simulink model "mdlref_paramargs"  (Simulink 6.0)
settings: Solver=FixedStepDiscrete  SolverMode=SingleTasking  StartTime=0.0  StopTime=10.0  FixedStep=0.1  RelTol=1e-3
undefined symbols (not defined in the file or in its folder): lower_saturation_limit, upper_saturation_limit
settings Model: Creator=The MathWorks Inc.  LastModifiedBy=batserve  ExtModeAutoUpdateStatusClock=off  ProdHWDeviceType=Specified
settings DataIOCC: SaveFormat=StructureWithTime  SignalLoggingName=logsOut
settings OptimizationCC: InlineParams=on
settings DebuggingCC: CheckExecutionContextPreStartOutputMsg=on  CheckExecutionContextRuntimeOutputMsg=on  SolverPrmCheckMsg=none
settings HardwareCC: ProdHWDeviceType=Specified  TargetHWDeviceType=32-bit Generic  ProdEqTarget=off
settings ModelReferenceCC: UpdateModelReferenceTargets=IfOutOfDate  CheckModelReferenceTargetMessage=none
settings RTWCC: GenerateReport=on  ProcessScript=grt_make_rtw_hook  LaunchReport=on

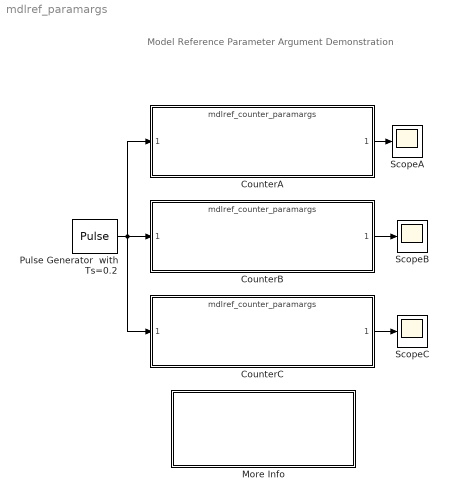
== system mdlref_paramargs ==
  note: Model Reference
      | Parameter Argument
      | Demonstration
  CounterA : ModelReference  ModelName=mdlref_counter_paramargs  ParameterArgumentNames=lower_saturation_limit,upper_saturation_limit  ParameterArgumentValues=0,20  ModelReferenceVersion=1.97  CopyOfModelName=mdlref_counter_paramargs
  CounterB : ModelReference  ModelName=mdlref_counter_paramargs  ParameterArgumentNames=lower_saturation_limit,upper_saturation_limit  ParameterArgumentValues=0,10  ModelReferenceVersion=1.97  CopyOfModelName=mdlref_counter_paramargs
  CounterC : ModelReference  ModelName=mdlref_counter_paramargs  ParameterArgumentNames=lower_saturation_limit,upper_saturation_limit  ParameterArgumentValues=0,5  ModelReferenceVersion=1.97  CopyOfModelName=mdlref_counter_paramargs
  More Info : Subsystem  PropExecContextAcrossSSBoundary=on
      settings: OpenFcn=mdlref_paramargsscript
      mask Display: disp('Double click here \nfor a step-by-step\ntutorial on this model')
  Pulse Generator  with Ts=0.2 : DiscretePulseGenerator  SampleTime=0.1  VectorParams1D=off
  ScopeA : Scope
      settings: TimeRange=10  YMin=-1  YMax=21  SaveName=ScopeDataA
  ScopeB : Scope
      settings: TimeRange=10  YMin=-1  YMax=21  SaveName=ScopeDataB
  ScopeC : Scope
      settings: TimeRange=10  YMin=-1  YMax=21  SaveName=ScopeDataC
  wires:
  CounterA/1 -> ScopeA/1
  Pulse Generator  with Ts=0.2/1 -> CounterB/1, CounterA/1, CounterC/1
  CounterC/1 -> ScopeC/1
  CounterB/1 -> ScopeB/1

== system mdlref_paramargs/More Info ==
  note: Bus Block Demonstration
  note: This demonstration shows how signals may be grouped and ungrouped while
      | retaining their names.  In this demonstration, 5 signals are created and labelled
      | appropriately.  These signals are then mux'd together to create a bus of signals.
      | This bus of signals is then fed into the Bus Selector block.  Inside of the Bus
      | Selector block, the Pulse and Chirp signals are chosen to be output from the
      | original signal bus.
      |
      | It is possible to place a nest signal buses and then still retrieve the original signal
      | with its label.
